simulink model "P4_ArduinoModel"  (R2024b)
settings: Solver=FixedStepDiscrete  StartTime=0.0  StopTime=Inf  FixedStep=0.01  RelTol=1e-3  EnableMultiTasking=on
PreLoadFcn:
  | path=uigetfile(pwd);
  | load(path)
  | gear_ratio=motor_param.gear_ratio;
undefined symbols (not defined in the file): motor_left, motor_param, motor_right
libraries: arduinolib x6, simulink x5, svdutilitieslib x4, slpidlib x2
settings Model: ExtModeTrigDuration=2  Creator=resjoehr  LastModifiedBy=resjoehr
settings SolverCC: AlgebraicLoopSolver=TrustRegion  AutoInsertRateTranBlk=on
settings DataIOCC: SaveFormat=Array  SaveOutput=off  SignalLogging=off  DSMLogging=off  SaveTime=off  ReturnWorkspaceOutputs=off
settings OptimizationCC: ReuseModelBlockBuffer=off  EnhancedBackFolding=on  PassReuseOutputArgsAs=Individual arguments  ZeroExternalMemoryAtStartup=off  ZeroInternalMemoryAtStartup=off  MaxStackSize=64  OptimizeBlockOrder=speed  DifferentSizesBufferReuse=on  EfficientTunableParamExpr=on
settings DebuggingCC: ParameterTunabilityLossMsg=error  UnconnectedInputMsg=warning  UnconnectedOutputMsg=warning  UnconnectedLineMsg=warning
settings HardwareCC: ProdBitPerInt=16  ProdBitPerPointer=16  ProdBitPerSizeT=16  ProdBitPerPtrDiffT=16  ProdLargestAtomicFloat=None  ProdWordSize=8  ProdHWDeviceType=Atmel->AVR
settings ModelReferenceCC: EnableRefExpFcnMdlSchedulingChecks=on
settings SFSimCC: MATLABDynamicMemAlloc=off
settings RTWCC: Description=Embedded Coder  SystemTargetFile=ert.tlc  HardwareBoard=Arduino Leonardo  TemplateMakefile=ert_default_tmf  GenerateReport=on  Toolchain=Arduino AVR  BuildConfiguration=Faster Runs  IncludeHyperlinkInReport=on  LaunchReport=on  GenerateTraceInfo=on  GenerateTraceReport=on  GenerateTraceReportSl=on  GenerateTraceReportSf=on  GenerateTraceReportEml=on  GPUComputeCapability=3.5  DLArmComputeVersion=19.05
settings CodeAppCC: ForceParamTrailComments=on  IgnoreCustomStorageClasses=off  OperatorAnnotations=on  SimulinkDataObjDesc=on  SFDataObjDesc=on  InsertBlockDesc=on
settings ERTTargetCC: SupportContinuousTime=on  SupportVariableSizeSignals=on  ExtModeStaticAllocSize=250  InlinedParameterPlacement=Hierarchical  DynamicArrayContainerType=coder::array

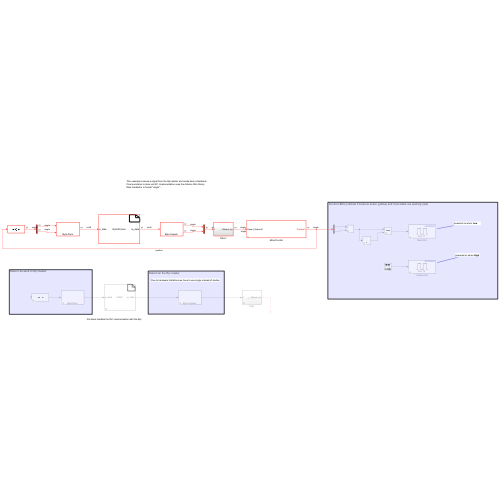
[thumbnail: Simulink's stored preview of the top-level diagram]
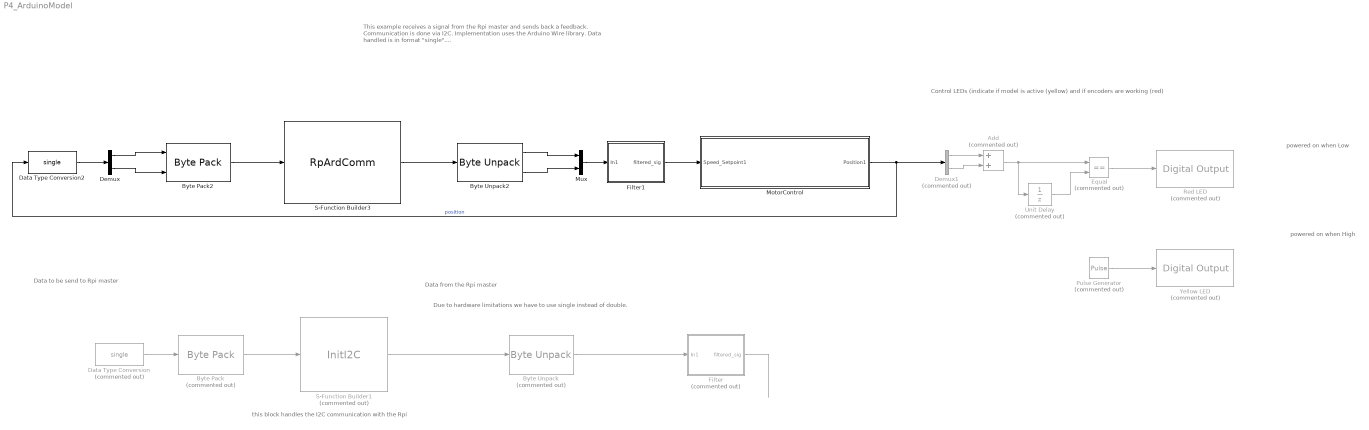
== system P4_ArduinoModel ==
  note: Control LEDs (indicate if model is active (yellow) and if encoders are working (red)
  note: Data to be send to Rpi master
  note: Data from the Rpi master
  note: this block handles the I2C communication with the Rpi
  note: Due to hardware limitations we have to use single instead of double.
  note: This example receives a signal from the Rpi master and sends back a feedback.
      | Communication is done via I2C. Implementation uses the Arduino Wire library.
      | Data handled is in format "single"....
  note: powered on when High
  note: powered on when Low
  Add : Sum  Commented=on
  Byte Pack : svdutilitieslib/Byte Pack  Commented=on  maskPackedDataType=uint8  datatypes={'single'}  byteAlign=1  blockPlatform=arduinoert
  Byte Pack2 : svdutilitieslib/Byte Pack  maskPackedDataType=uint8  datatypes={'single','single'}  byteAlign=1  blockPlatform=arduinoert
  Byte Unpack : svdutilitieslib/Byte Unpack  Commented=on  dimensions={[1]}  datatypes={'single'}  byteAlign=1  blockPlatform=arduinoert
  Byte Unpack2 : svdutilitieslib/Byte Unpack  dimensions={[1],[1]}  datatypes={'single','single'}  byteAlign=1  blockPlatform=arduinoert
  Data Type Conversion : DataTypeConversion  Commented=on  OutDataTypeStr=single  SaturateOnIntegerOverflow=off  RndMeth=Floor
  Data Type Conversion2 : DataTypeConversion  OutDataTypeStr=single  SaturateOnIntegerOverflow=off  RndMeth=Floor
  Demux : Demux  Outputs=2
  Demux1 : Demux  Commented=on  Outputs=2
  Equal : RelationalOperator  Commented=on  Operator===  OutDataTypeStr=boolean  RndMeth=Simplest  InputSameDT=off
  Filter : Subsystem  Commented=on
  Filter1 : Subsystem
  MotorControl : Subsystem  mask{motor_gear=motor_param.motor_ratio, gear_box=gear_ratio}
      mask prompts: motor_gear "Motor gear ratio:"; gear_box "Gear box ratio:"
      mask DialogControl DescTextVar Prompt: Please specify the parameters of the gears. This is required to translate the encoder signal to the angular velocity of the wheels. The ratio has to be entered as a double. I.e. 49:17=2.88.
      mask DialogControl ParameterGroupVar Prompt: Gear Box Parameters
  Mux : Mux  Inputs=2
  Pulse Generator : DiscretePulseGenerator  Commented=on  Period=500  PulseWidth=250  SampleTime=-1
  Red LED : arduinolib/Digital Output  Commented=on  pinNumber=17  Direction=output  blockPlatform=arduino
  S-Function Builder1 : S-Function  Commented=on  InitFcn=try, set_param(gcb,'FunctionName','InitI2C'), end  FunctionName=InitI2C  Parameters=uint8(7)  SFunctionModules=InitI2C_wrapper.cpp  SFunctionDeploymentMode=off  EnableBusSupport=off  mask(S-Function Builder){}
      mask help: Simulink:masks:SFunctionBuilder_MD
      mask init:
      | val = [[.9  0.75 0.75 1 1 .9 .9 1]',[1 1 0.75 0.75 .9 .9 1 .9]'];try , sys = get_param(gcb,'SfunBuilderFcnName');if isempty(sys), sys = get_param(gcb,'FunctionName'); end,catch, sys = get_param(gcb,'FunctionName'); end
      settings: CopyFcn=set_param(gcbh,'LinkStatus','none')  PreSaveFcn=try, set_param(gcb,'FunctionName','InitI2C'), end  OpenFcn=sfunctionwizard(gcbh)
      mask Display:
      | plot(val(:,1),val(:,2))
      | disp(sys)
      | port_label('input',1,'a_data')
      | port_label('output',1,'rp_data')
  S-Function Builder3 : S-Function  FunctionName=RpArdComm  Parameters=uint8(7)  SFunctionModules=RpArdComm_wrapper.cpp  SFunctionDeploymentMode=off  EnableBusSupport=off  mask(S-Function Builder){}
      mask help: Simulink:masks:SFunctionBuilder_MD
      mask init: same as P4_ArduinoModel/S-Function Builder1
      settings: CopyFcn=set_param(gcbh,'LinkStatus','none')  OpenFcn=sfunctionwizard(gcbh)
      mask Display:
      | plot(val(:,1),val(:,2))
      | disp(sys)
      | port_label('input',1,sprintf('%s', 'a\_data'),'interpreter','tex')
      | port_label('output',1,sprintf('%s', 'rp\_data'),'interpreter','tex')
  Unit Delay : UnitDelay  Commented=on  SampleTime=-1  HasFrameUpgradeWarning=on
  Yellow LED : arduinolib/Digital Output  Commented=on  pinNumber=13  Direction=output  blockPlatform=arduino
  wires:
  Byte Pack/1 -> S-Function Builder1/1
  MotorControl/1(Position1) -> Data Type Conversion2/1, Demux1/1  "position"
  Data Type Conversion/1 -> Byte Pack/1
  S-Function Builder1/1 -> Byte Unpack/1
  Byte Unpack/1 -> Filter/1(In1)
  Filter/1(filtered_sig) -> ?
  S-Function Builder3/1 -> Byte Unpack2/1
  Byte Pack2/1 -> S-Function Builder3/1
  Demux/1 -> Byte Pack2/1
  Demux/2 -> Byte Pack2/2
  Mux/1 -> Filter1/1(In1)
  Byte Unpack2/1 -> Mux/1
  Byte Unpack2/2 -> Mux/2
  Filter1/1(filtered_sig) -> MotorControl/1(Speed_Setpoint1)
  Data Type Conversion2/1 -> Demux/1
  Pulse Generator/1 -> Yellow LED/1
  Unit Delay/1 -> Equal/2
  Equal/1 -> Red LED/1
  Demux1/1 -> Add/1
  Demux1/2 -> Add/2
  Add/1 -> Unit Delay/1, Equal/1

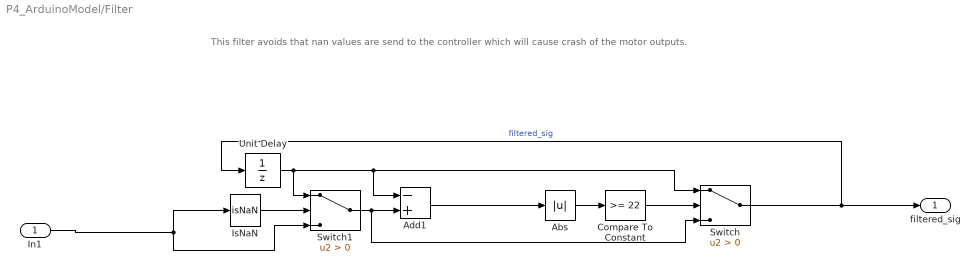
== system P4_ArduinoModel/Filter ==
  note: This filter avoids that nan values are send to the controller which will cause crash of the motor outputs.
  In1 : Inport
  Abs : Abs  SaturateOnIntegerOverflow=off
  Add1 : Sum  Inputs=-+
  Compare To Constant : simulink/Logic and Bit Operations/Compare To Constant  relop=>=  const=22  OutDataTypeStr=boolean
  IsNaN : RelationalOperator  Operator=isNaN  OutDataTypeStr=boolean  RndMeth=Simplest  InputSameDT=off
  Switch : Switch  Criteria=u2 > Threshold  SaturateOnIntegerOverflow=off  InputSameDT=off
  Switch1 : Switch  Criteria=u2 > Threshold  SaturateOnIntegerOverflow=off  InputSameDT=off
  Unit Delay : UnitDelay  SampleTime=-1  HasFrameUpgradeWarning=on
  filtered_sig : Outport
  wires:
  IsNaN/1 -> Switch1/2
  Switch1/1 -> Add1/2, Switch/3
  Switch/1 -> filtered_sig/1, Unit Delay/1  "filtered_sig"
  In1/1 -> IsNaN/1, Switch1/3
  Abs/1 -> Compare To Constant/1
  Compare To Constant/1 -> Switch/2
  Unit Delay/1 -> Switch/1, Add1/1, Switch1/1
  Add1/1 -> Abs/1

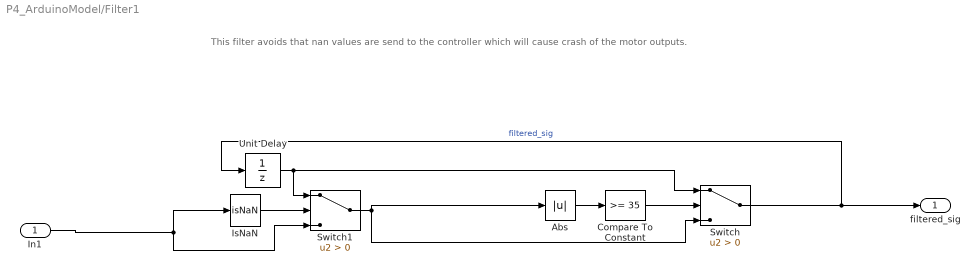
== system P4_ArduinoModel/Filter1 ==
  note: This filter avoids that nan values are send to the controller which will cause crash of the motor outputs.
  In1 : Inport
  Abs : Abs  SaturateOnIntegerOverflow=off
  Compare To Constant : simulink/Logic and Bit Operations/Compare To Constant  relop=>=  const=35  OutDataTypeStr=boolean
  IsNaN : RelationalOperator  Operator=isNaN  OutDataTypeStr=boolean  RndMeth=Simplest  InputSameDT=off
  Switch : Switch  Criteria=u2 > Threshold  SaturateOnIntegerOverflow=off  InputSameDT=off
  Switch1 : Switch  Criteria=u2 > Threshold  SaturateOnIntegerOverflow=off  InputSameDT=off
  Unit Delay : UnitDelay  SampleTime=-1  HasFrameUpgradeWarning=on
  filtered_sig : Outport
  wires:
  IsNaN/1 -> Switch1/2
  Switch/1 -> filtered_sig/1, Unit Delay/1  "filtered_sig"
  In1/1 -> IsNaN/1, Switch1/3
  Abs/1 -> Compare To Constant/1
  Compare To Constant/1 -> Switch/2
  Unit Delay/1 -> Switch/1, Switch1/1
  Switch1/1 -> Abs/1, Switch/3

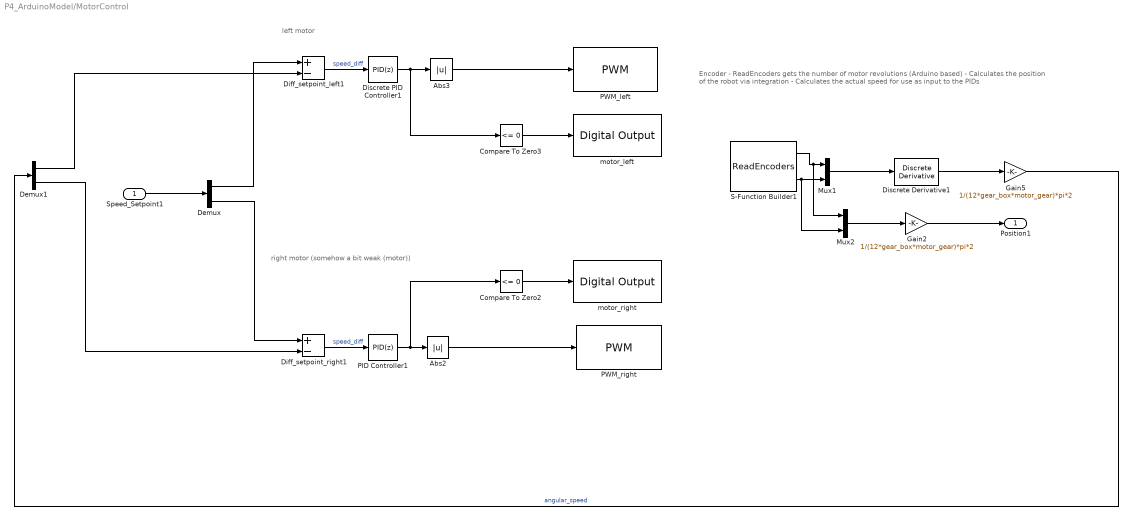
== system P4_ArduinoModel/MotorControl ==
  note: Encoder
      | - ReadEncoders gets the number of motor revolutions (Arduino based)
      | - Calculates the position of the robot via integration
      | - Calculates the actual speed for use as input to the PIDs
  note: left motor
  note: right motor
      | (somehow a bit weak (motor))
  Speed_Setpoint1 : Inport  OutDataTypeStr=single  SampleTime=0.01
  Abs2 : Abs  SaturateOnIntegerOverflow=off
  Abs3 : Abs  SaturateOnIntegerOverflow=off  OutDataTypeStr=Inherit: Inherit via internal rule
  Compare To Zero2 : simulink/Logic and Bit Operations/Compare To Zero  relop=<=  OutDataTypeStr=boolean
  Compare To Zero3 : simulink/Logic and Bit Operations/Compare To Zero  relop=<=  OutDataTypeStr=boolean
  Demux : Demux  Outputs=2
  Demux1 : Demux  Outputs=2
  Diff_setpoint_left1 : Sum  Inputs=+-
  Diff_setpoint_right1 : Sum  Inputs=+-
  Discrete Derivative1 : simulink/Discrete/Discrete Derivative  gainval=1  ICPrevScaledInput=0.0  OutMin=[]  OutMax=[]  OutDataType=fixdt(1, 16)  OutScaling=2^-10  DoSatur=off
  Discrete PID Controller1 : slpidlib/PID Controller  Controller=PID  Form=Parallel  TimeDomain=Discrete-time  UseExternalTs=off  SampleTime=0.01  IntegratorMethod=Forward Euler  FilterMethod=Forward Euler  ControllerParametersSource=internal  P=motor_left.P  I=motor_left.I  UseKiTs=off  D=motor_left.D  UseExternalDerivativeSource=off  N=motor_left.N  UseFilter=on  TunerSelectOption=Transfer Function Based (PID Tuner App)  InitialConditionSource=internal  InitialConditionForIntegrator=0  InitialConditionForFilter=0  DifferentiatorICPrevScaledInput=0  ExternalReset=none  TrackingMode=off  Kt=1  LimitOutput=on  SatLimitsSource=internal  UpperSaturationLimit=250  LowerSaturationLimit=-250  LinearizeAsGain=off  AntiWindupMode=clamping  Kb=1  LimitIntegrator=off  UpperIntegratorSaturationLimit=inf  LowerIntegratorSaturationLimit=-inf  POutMin=[]  POutMax=[]  IOutMin=[]  IOutMax=[]  DOutMin=[]  DOutMax=[]  NOutMin=[]  NOutMax=[]  SumOutMin=[]  SumOutMax=[]  SaturationOutMin=[]  SaturationOutMax=[]  PParamMin=[]  PParamMax=[]  IParamMin=[]  IParamMax=[]  DParamMin=[]  DParamMax=[]  NParamMin=[]  NParamMax=[]  KbParamMin=[]  KbParamMax=[]  KtParamMin=[]  KtParamMax=[]  KbOutMin=[]  KbOutMax=[]  KtOutMin=[]  KtOutMax=[]  IntegratorOutMin=[]  IntegratorOutMax=[]  FilterOutMin=[]  FilterOutMax=[]  SumI1OutMin=[]  SumI1OutMax=[]  SumI2OutMin=[]  SumI2OutMax=[]  SumI3OutMin=[]  SumI3OutMax=[]  SumI4OutMin=[]  SumI4OutMax=[]  SumDOutMin=[]  SumDOutMax=[]  DifferentiatorOutMin=[]  DifferentiatorOutMax=[]  FilterDiffOutCoefMin=[]  FilterDiffOutCoefMax=[]  ReciprocalOutMin=[]  ReciprocalOutMax=[]  SumDenOutMin=[]  SumDenOutMax=[]  SumNumOutMin=[]  SumNumOutMax=[]  DivideOutMin=[]  DivideOutMax=[]  UdiffTsProdOutMin=[]  UdiffTsProdOutMax=[]  NTsProdOutMin=[]  NTsProdOutMax=[]  UintegralTsProdOutMin=[]  UintegralTsProdOutMax=[]  UngainTsProdOutMin=[]  UngainTsProdOutMax=[]  ClampingZeroOutDataTypeStr=Inherit: Inherit via back propagation  ClampingZeroOutMin=[]  ClampingZeroOutMax=[]  FilterDenConstantOutDataTypeStr=Inherit: Inherit via back propagation  FilterDenConstantOutMin=[]  FilterDenConstantOutMax=[]  PCopyOutDataTypeStr=Inherit: Inherit via back propagation  PCopyOutMin=[]  PCopyOutMax=[]  NCopyOutDataTypeStr=Inherit: Inherit via back propagation  NCopyOutMin=[]  NCopyOutMax=[]  IntegratorContinuousStateAttributes=''  IntegratorStateMustResolveToSignalObject=off  IntegratorRTWStateStorageClass=Auto  FilterContinuousStateAttributes=''  FilterStateMustResolveToSignalObject=off  FilterRTWStateStorageClass=Auto  ParallelPVariant=InternalParameters  IdealPVariant=Disabled  IVariant=InternalParameters  DVariant=InternalParameters  IntegratorVariant=Discrete  SatVariant=Enabled  AWVariant=DiscClampingParallel  PCopyVariant=Disabled  TRVariant=Disabled  FdbkBlocksVariant=Forward  IdealPFdbkVariant=Disabled  SatFdbkVariant=Disabled  DerivativeFilterVariant=ForwardEulerFilter  NVariant=InternalParameters  NCopyVariant=Disabled  FilterICVariant=InternalICsFilter  IntegratorICVariant=InternalICs  ExternalResetVariant=Disabled  TRSumVariant=Passthrough  SumFdbkVariant=Disabled  SumVariant=Sum_PID  TsampFilterVariant=InternalTs  TsampNgainVariant=Passthrough  TsampIntegralVariant=Disabled_SignalSpec  ExternalSaturationOutDataTypeStr=Inherit: Same as second input  DerivativeSourceVariant=ErrorSignal  PreIntVariant=InternalPreInt
  Gain2 : Gain  Gain=1/(12*gear_box*motor_gear)*pi*2  OutDataTypeStr=single
  Gain5 : Gain  Gain=1/(12*gear_box*motor_gear)*pi*2
  Mux1 : Mux  Inputs=2
  Mux2 : Mux  Inputs=2
  PID Controller1 : slpidlib/PID Controller  Controller=PID  Form=Parallel  TimeDomain=Discrete-time  UseExternalTs=off  SampleTime=0.01  IntegratorMethod=Forward Euler  FilterMethod=Forward Euler  ControllerParametersSource=internal  P=motor_right.P  I=motor_right.I  UseKiTs=off  D=motor_right.D  UseExternalDerivativeSource=off  N=motor_right.N  UseFilter=on  TunerSelectOption=Transfer Function Based (PID Tuner App)  InitialConditionSource=internal  InitialConditionForIntegrator=0  InitialConditionForFilter=0  DifferentiatorICPrevScaledInput=0  ExternalReset=none  TrackingMode=off  Kt=1  LimitOutput=on  SatLimitsSource=internal  UpperSaturationLimit=250  LowerSaturationLimit=-250  LinearizeAsGain=on  AntiWindupMode=clamping  Kb=1  LimitIntegrator=off  UpperIntegratorSaturationLimit=inf  LowerIntegratorSaturationLimit=-inf  POutMin=[]  POutMax=[]  IOutMin=[]  IOutMax=[]  DOutMin=[]  DOutMax=[]  NOutMin=[]  NOutMax=[]  SumOutMin=[]  SumOutMax=[]  SaturationOutMin=[]  SaturationOutMax=[]  PParamMin=[]  PParamMax=[]  IParamMin=[]  IParamMax=[]  DParamMin=[]  DParamMax=[]  NParamMin=[]  NParamMax=[]  KbParamMin=[]  KbParamMax=[]  KtParamMin=[]  KtParamMax=[]  KbOutMin=[]  KbOutMax=[]  KtOutMin=[]  KtOutMax=[]  IntegratorOutMin=[]  IntegratorOutMax=[]  FilterOutMin=[]  FilterOutMax=[]  SumI1OutMin=[]  SumI1OutMax=[]  SumI2OutMin=[]  SumI2OutMax=[]  SumI3OutMin=[]  SumI3OutMax=[]  SumI4OutMin=[]  SumI4OutMax=[]  SumDOutMin=[]  SumDOutMax=[]  DifferentiatorOutMin=[]  DifferentiatorOutMax=[]  FilterDiffOutCoefMin=[]  FilterDiffOutCoefMax=[]  ReciprocalOutMin=[]  ReciprocalOutMax=[]  SumDenOutMin=[]  SumDenOutMax=[]  SumNumOutMin=[]  SumNumOutMax=[]  DivideOutMin=[]  DivideOutMax=[]  UdiffTsProdOutMin=[]  UdiffTsProdOutMax=[]  NTsProdOutMin=[]  NTsProdOutMax=[]  UintegralTsProdOutMin=[]  UintegralTsProdOutMax=[]  UngainTsProdOutMin=[]  UngainTsProdOutMax=[]  ClampingZeroOutDataTypeStr=Inherit: Inherit via back propagation  ClampingZeroOutMin=[]  ClampingZeroOutMax=[]  FilterDenConstantOutDataTypeStr=Inherit: Inherit via back propagation  FilterDenConstantOutMin=[]  FilterDenConstantOutMax=[]  PCopyOutDataTypeStr=Inherit: Inherit via back propagation  PCopyOutMin=[]  PCopyOutMax=[]  NCopyOutDataTypeStr=Inherit: Inherit via back propagation  NCopyOutMin=[]  NCopyOutMax=[]  IntegratorContinuousStateAttributes=''  IntegratorStateMustResolveToSignalObject=off  IntegratorRTWStateStorageClass=Auto  FilterContinuousStateAttributes=''  FilterStateMustResolveToSignalObject=off  FilterRTWStateStorageClass=Auto  ParallelPVariant=InternalParameters  IdealPVariant=Disabled  IVariant=InternalParameters  DVariant=InternalParameters  IntegratorVariant=Discrete  SatVariant=Enabled  AWVariant=DiscClampingParallel  PCopyVariant=Disabled  TRVariant=Disabled  FdbkBlocksVariant=Forward  IdealPFdbkVariant=Disabled  SatFdbkVariant=Disabled  DerivativeFilterVariant=ForwardEulerFilter  NVariant=InternalParameters  NCopyVariant=Disabled  FilterICVariant=InternalICsFilter  IntegratorICVariant=InternalICs  ExternalResetVariant=Disabled  TRSumVariant=Passthrough  SumFdbkVariant=Disabled  SumVariant=Sum_PID  TsampFilterVariant=InternalTs  TsampNgainVariant=Passthrough  TsampIntegralVariant=Disabled_SignalSpec  ExternalSaturationOutDataTypeStr=Inherit: Same as second input  DerivativeSourceVariant=ErrorSignal  PreIntVariant=InternalPreInt
  PWM_left : arduinolib/PWM  pinNumber=motor_left.PWMpin  frequencyType=Default  desiredFrequency=5000  achievableFrequency=5000
  PWM_right : arduinolib/PWM  pinNumber=motor_right.PWMpin  frequencyType=Default  desiredFrequency=5000  achievableFrequency=5000
  S-Function Builder1 : S-Function  InitFcn=try, set_param(gcb,'FunctionName','ReadEncoders'), end  FunctionName=ReadEncoders  SFunctionModules=ReadEncoders_wrapper.cpp  SFunctionDeploymentMode=off  EnableBusSupport=off  mask(S-Function Builder){}
      mask help: Simulink:masks:SFunctionBuilder_MD
      mask init: same as P4_ArduinoModel/S-Function Builder1
      settings: CopyFcn=set_param(gcbh,'LinkStatus','none')  PreSaveFcn=try, set_param(gcb,'FunctionName','ReadEncoders'), end  OpenFcn=sfunctionwizard(gcbh)
      mask Display:
      | plot(val(:,1),val(:,2))
      | disp(sys)
      | port_label('output',1,'left')
      | port_label('output',2,'right')
  motor_left : arduinolib/Digital Output  pinNumber=motor_left.Pin  Direction=output  blockPlatform=arduino
  motor_right : arduinolib/Digital Output  pinNumber=motor_right.Pin  Direction=output  blockPlatform=arduino
  Position1 : Outport  OutDataTypeStr=single
  wires:
  Compare To Zero3/1 -> motor_left/1
  PID Controller1/1 -> Abs2/1, Compare To Zero2/1
  Diff_setpoint_left1/1 -> Discrete PID Controller1/1  "speed_diff"
  Discrete PID Controller1/1 -> Abs3/1, Compare To Zero3/1
  S-Function Builder1/1 -> Mux2/1, Mux1/1
  Gain2/1 -> Position1/1
  Demux1/1 -> Diff_setpoint_left1/2
  Demux/1 -> Diff_setpoint_left1/1
  Demux1/2 -> Diff_setpoint_right1/2
  Discrete Derivative1/1 -> Gain5/1
  S-Function Builder1/2 -> Mux2/2, Mux1/2
  Mux2/1 -> Gain2/1
  Mux1/1 -> Discrete Derivative1/1
  Compare To Zero2/1 -> motor_right/1
  Gain5/1 -> Demux1/1  "angular_speed"
  Diff_setpoint_right1/1 -> PID Controller1/1  "speed_diff"
  Speed_Setpoint1/1 -> Demux/1
  Demux/2 -> Diff_setpoint_right1/1
  Abs3/1 -> PWM_left/1
  Abs2/1 -> PWM_right/1
